simulink model "sens_example_pendulum_sim"  (R2017a)
settings: Solver=ode5  StartTime=0.0  StopTime=30  FixedStep=0.01  MaxStep=0.01  RelTol=1e-3  EnableMultiTasking=on
model workspace (MAT data in the model file):
  f = 0.69
  g = 9.78
  l = 1.3
  m = 2.4
  p = [2.80579193708; 1.4882371127; 9.68918520433; 0.661909970783]
  par = [2.32143588587; 1.10554303073; 9.72701226611; 0.702090686836]
settings Model: Creator=Carlos Mario  LastModifiedBy=drojasd
settings DataIOCC: SaveFormat=Array  SignalLogging=off  DSMLogging=off  ReturnWorkspaceOutputs=on  OutputTimes=tout
settings OptimizationCC: LifeSpan=inf
settings DebuggingCC: UnderspecifiedInitializationDetection=Classic  MergeDetectMultiDrivingBlocksExec=none  SolverPrmCheckMsg=warning  StateNameClashWarn=warning  SFUnexpectedBacktrackingDiag=warning  SFNoUnconditionalDefaultTransitionDiag=warning  SFExecutionAtInitializationDiag=none
settings HardwareCC: ProdBitPerPointer=32  ProdBitPerSizeT=32  ProdBitPerPtrDiffT=32  ProdLargestAtomicFloat=None  ProdIntDivRoundTo=Undefined  ProdEndianess=Unspecified  ProdWordSize=32  ProdHWDeviceType=32-bit Generic
settings ModelReferenceCC: PropagateSignalLabelsOutOfModel=off
settings GRTTargetCC: TargetLangStandard=C89/C90 (ANSI)  GeneratePreprocessorConditionals=Disable all
settings ConfigComp: CovMetricSettings=dw  CovHtmlReporting=on  CovSaveCumulativeToWorkspaceVar=on  CovSaveSingleToWorkspaceVar=on  CovExternalEMLEnable=off

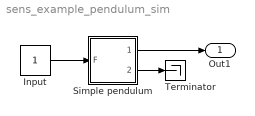
== system sens_example_pendulum_sim ==
  Input : Constant
  Simple pendulum : Subsystem  mask(Mathematical model){par=[m l g f], x0=[pi/4 0]}
      mask prompts: par "[m l g f]"; x0 "Initial conditions (th0, omega0)"
      mask help: Simple pendulum
      mask init:
      | m=par(1); l=par(2); g=par(3); f=par(4);
      mask Display: plot([.1,.9],[.9,.9],[.5,.2],[.9,.25],[.475,.475,.525,.525,.475],[.875,.925,.925,.875,.875])
  Terminator : Terminator
  Out1 : Outport
  wires:
  Simple pendulum/1(theta) -> Out1/1
  Simple pendulum/2(theta') -> Terminator/1
  Input/1 -> Simple pendulum/1(F)

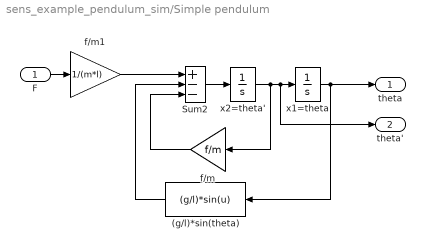
== system sens_example_pendulum_sim/Simple pendulum ==
  F : Inport
  (g/l)*sin(theta) : Fcn  Expr=(g/l)*sin(u)
  Sum2 : Sum  Inputs=+--  SaturateOnIntegerOverflow=on  InputSameDT=on  OutDataTypeStr=Inherit: Same as first input
  f/m : Gain  Gain=f/m  SaturateOnIntegerOverflow=on  OutDataTypeStr=Inherit: Same as input  ParamDataTypeStr=Inherit: Same as input
  f/m1 : Gain  Gain=1/(m*l)  SaturateOnIntegerOverflow=on  OutDataTypeStr=Inherit: Same as input  ParamDataTypeStr=Inherit: Same as input
  x1=theta : Integrator  InitialCondition=x0(1)
  x2=theta' : Integrator  InitialCondition=x0(2)
  theta : Outport
  theta' : Outport  Port=2
  wires:
  F/1 -> f/m1/1
  (g/l)*sin(theta)/1 -> Sum2/2
  x1=theta/1 -> theta/1, (g/l)*sin(theta)/1
  x2=theta'/1 -> theta'/1, x1=theta/1, f/m/1
  f/m/1 -> Sum2/3
  Sum2/1 -> x2=theta'/1
  f/m1/1 -> Sum2/1
